simulink model "Simulink_1"  (R2023b)
settings: Solver=FixedStepAuto  StartTime=0.0  StopTime=T  FixedStep=step_size  RelTol=1e-6  AbsTol=1e-6
values from neighbouring files (symbols this model uses):
  A_in = scales(NN)    [synthetic_data.m]
  Dth0 = 0    [synthetic_data.m]
  Kf = 0.001    [synthetic_data.m]
  Om_in = input_freq(NN)    [synthetic_data.m]
  p1 = params(1)    [butterfly_real_data.m]    (also in synthetic_data.m)
  p2 = params(2)    [butterfly_real_data.m]    (also in synthetic_data.m)
  p3 = params(3)    [butterfly_real_data.m]    (also in synthetic_data.m)
  th0 = 0.01    [synthetic_data.m]
libraries: simulink x2
settings Model: Creator=shiriaev  LastModifiedBy=Artem
settings SolverCC: AlgebraicLoopSolver=TrustRegion
settings DebuggingCC: UnconnectedInputMsg=warning  UnconnectedOutputMsg=warning  UnconnectedLineMsg=warning
settings ModelReferenceCC: EnableRefExpFcnMdlSchedulingChecks=on

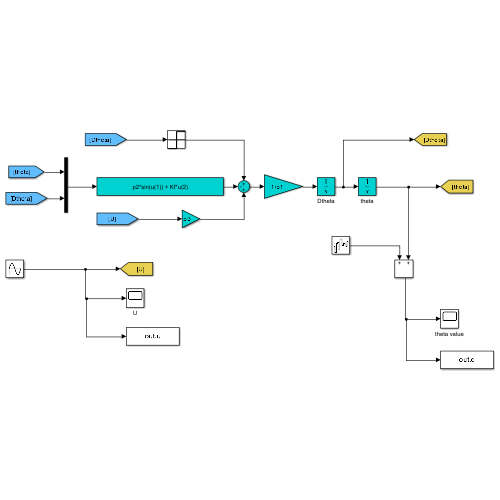
[thumbnail: Simulink's stored preview of the top-level diagram]
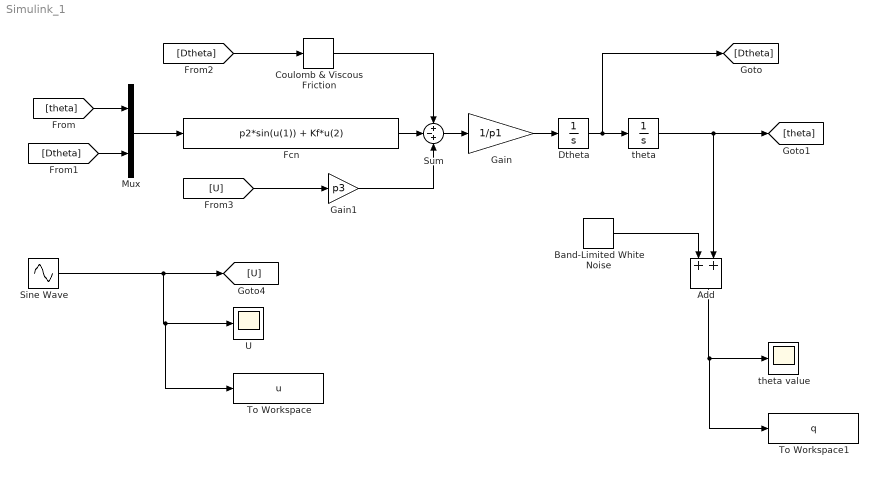
== system Simulink_1 ==
  Add : Sum
  Band-Limited White Noise : simulink/Sources/Band-Limited White Noise  Cov=[0.00000001]  Ts=0.01  seed=seed_rand
  Coulomb & Viscous Friction : simulink/Discontinuities/Coulomb & Viscous Friction  offset=0.00000005  gain=0
  Dtheta : Integrator  InitialCondition=Dth0
  Fcn : Fcn  Expr=p2*sin(u(1)) + Kf*u(2)
  Gain : Gain  Gain=1/p1
  Gain1 : Gain  Gain=p3
  Mux : Mux  Inputs=2
  Sine Wave : Sin  Amplitude=A_in  Frequency=Om_in  SampleTime=0
  Sum : Sum  Inputs=+-+
  To Workspace : ToWorkspace  VariableName=u  SaveFormat=Timeseries  SampleTime=-1
  To Workspace1 : ToWorkspace  VariableName=q  SaveFormat=Timeseries  SampleTime=-1
  U : Scope
  theta : Integrator  InitialCondition=th0
  theta value : Scope
  wires:
  Dtheta/1 -> [Dtheta], theta/1
  theta/1 -> Add/2, [theta]
  [theta] -> Mux/1
  [Dtheta] -> Mux/2
  Mux/1 -> Fcn/1
  Gain/1 -> Dtheta/1
  Sum/1 -> Gain/1
  [U] -> Gain1/1
  Sine Wave/1 -> To Workspace/1, U/1, [U]
  [Dtheta] -> Coulomb & Viscous Friction/1
  Coulomb & Viscous Friction/1 -> Sum/1
  Fcn/1 -> Sum/2
  Gain1/1 -> Sum/3
  Band-Limited White Noise/1 -> Add/1
  Add/1 -> To Workspace1/1, theta value/1
